simulink model "evaluateDis"  (R2016b)
settings: Solver=VariableStepAuto  StartTime=0.0  StopTime=0.4  RelTol=1e-3
values from neighbouring files (symbols this model uses):
  plant = tf(1,[0.01 1])    [transferfunDisObserver_sim.m]
settings Model: Creator=Yu  LastModifiedBy=Yu

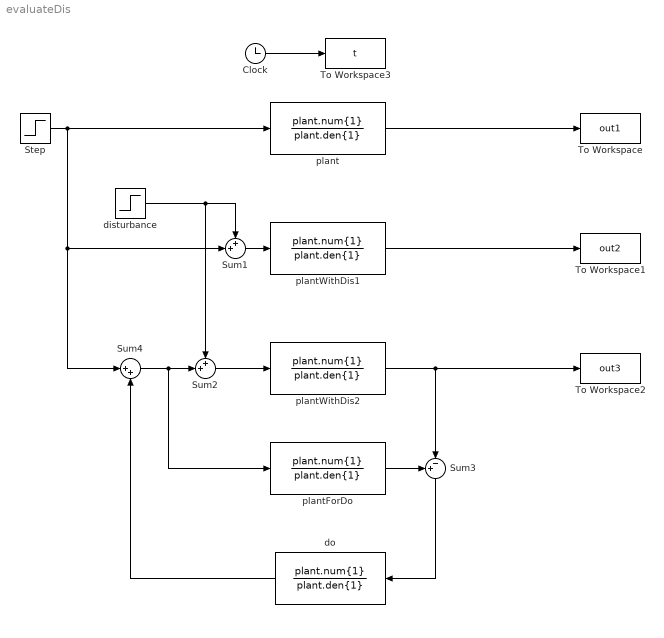
== system evaluateDis ==
  Clock : Clock
  Step : Step  Time=0.01  SampleTime=0
  Sum1 : Sum  Inputs=++|
  Sum2 : Sum  Inputs=++|
  Sum3 : Sum  Inputs=+-|
  Sum4 : Sum  Inputs=|++
  To Workspace : ToWorkspace  VariableName=out1  SampleTime=-1
  To Workspace1 : ToWorkspace  VariableName=out2  SampleTime=-1
  To Workspace2 : ToWorkspace  VariableName=out3  SampleTime=-1
  To Workspace3 : ToWorkspace  VariableName=t  SampleTime=-1
  disturbance : Step  Time=0.2  After=0.3  SampleTime=0
  do : TransferFcn  Numerator=plant.num{1}  Denominator=plant.den{1}
  plant : TransferFcn  Numerator=plant.num{1}  Denominator=plant.den{1}
  plantForDo : TransferFcn  Numerator=plant.num{1}  Denominator=plant.den{1}
  plantWithDis1 : TransferFcn  Numerator=plant.num{1}  Denominator=plant.den{1}
  plantWithDis2 : TransferFcn  Numerator=plant.num{1}  Denominator=plant.den{1}
  wires:
  Step/1 -> plant/1, Sum4/1, Sum1/2
  Sum1/1 -> plantWithDis1/1
  Sum2/1 -> plantWithDis2/1
  disturbance/1 -> Sum2/1, Sum1/1
  plantForDo/1 -> Sum3/1
  plantWithDis2/1 -> To Workspace2/1, Sum3/2
  Sum3/1 -> do/1
  Sum4/1 -> plantForDo/1, Sum2/2
  do/1 -> Sum4/2
  plant/1 -> To Workspace/1
  plantWithDis1/1 -> To Workspace1/1
  Clock/1 -> To Workspace3/1
